simulink model "assignmen4"  (R2017a)
settings: Solver=VariableStepAuto  StartTime=0.0  StopTime=10.0  RelTol=1e-3
libraries: simulink x12, hdlsllib x12
settings Model: Creator=zhao.yi4  LastModifiedBy=yaleduffy
settings OptimizationCC: BlockReduction=off  ConditionallyExecuteInputs=off  DefaultParameterBehavior=Inlined
settings DebuggingCC: AlgebraicLoopMsg=error
settings HardwareCC: ProdBitPerPointer=32  ProdBitPerSizeT=32  ProdBitPerPtrDiffT=32  ProdLargestAtomicFloat=None  ProdIntDivRoundTo=Undefined  ProdEndianess=Unspecified  ProdWordSize=32  ProdHWDeviceType=ASIC/FPGA->ASIC/FPGA  ProdEqTarget=off

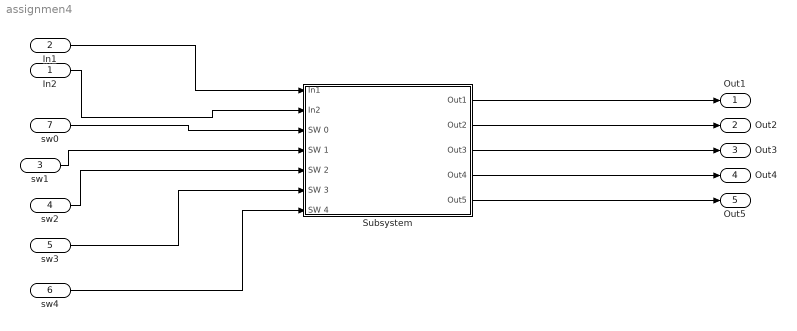
== system assignmen4 ==
  In2 : Inport  OutDataTypeStr=boolean  SampleTime=1
  In1 : Inport  Port=2  OutDataTypeStr=boolean  SampleTime=1
  sw1 : Inport  Port=3  OutDataTypeStr=boolean  SampleTime=1
  sw2 : Inport  Port=4  OutDataTypeStr=boolean  SampleTime=1
  sw3 : Inport  Port=5  OutDataTypeStr=boolean  SampleTime=1
  sw4 : Inport  Port=6  OutDataTypeStr=boolean  SampleTime=1
  sw0 : Inport  Port=7  OutDataTypeStr=boolean  SampleTime=1
  Subsystem : Subsystem
  Out1 : Outport
  Out2 : Outport  Port=2
  Out3 : Outport  Port=3
  Out4 : Outport  Port=4
  Out5 : Outport  Port=5
  wires:
  In2/1 -> Subsystem/2(In2)
  Subsystem/1(Out1) -> Out1/1
  In1/1 -> Subsystem/1(In1)
  sw2/1 -> Subsystem/5(SW 2)
  sw3/1 -> Subsystem/6(SW 3)
  sw4/1 -> Subsystem/7(SW 4)
  sw1/1 -> Subsystem/4(SW 1)
  sw0/1 -> Subsystem/3(SW 0)
  Subsystem/2(Out2) -> Out2/1
  Subsystem/3(Out3) -> Out3/1
  Subsystem/4(Out4) -> Out4/1
  Subsystem/5(Out5) -> Out5/1

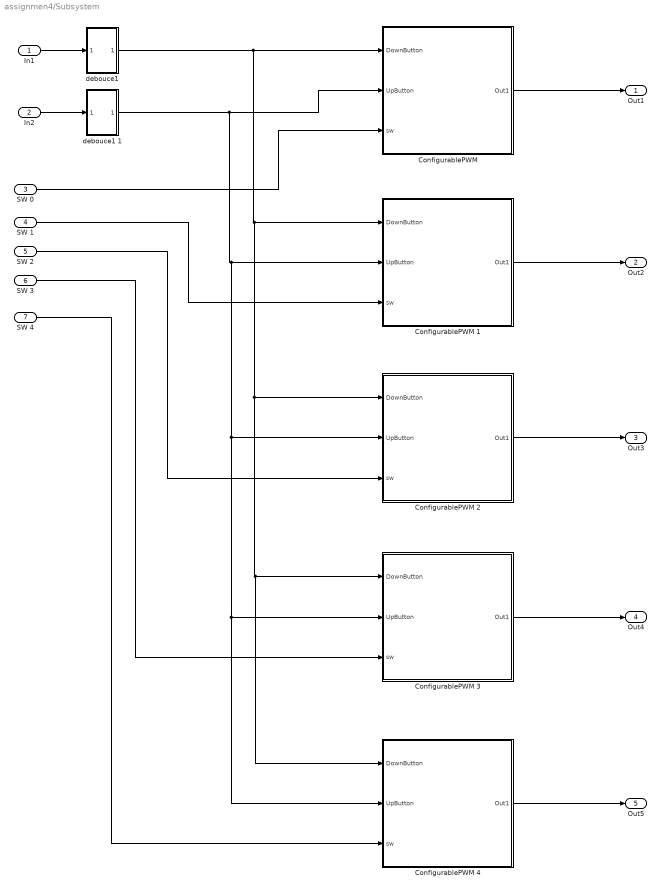
== system assignmen4/Subsystem ==
  In1 : Inport  OutDataTypeStr=boolean  SampleTime=1
  In2 : Inport  Port=2  OutDataTypeStr=boolean  SampleTime=1
  SW 0 : Inport  Port=3  OutDataTypeStr=boolean  SampleTime=1
  SW 1 : Inport  Port=4  OutDataTypeStr=boolean  SampleTime=1
  SW 2 : Inport  Port=5  OutDataTypeStr=boolean  SampleTime=1
  SW 3 : Inport  Port=6  OutDataTypeStr=boolean  SampleTime=1
  SW 4 : Inport  Port=7  OutDataTypeStr=boolean  SampleTime=1
  "ConfigurablePWM " : Subsystem
  ConfigurablePWM 1 : Subsystem
  ConfigurablePWM 2 : Subsystem
  ConfigurablePWM 3 : Subsystem
  ConfigurablePWM 4 : Subsystem
  "debouce1 " : Subsystem
  debouce1 1 : Subsystem
  Out1 : Outport
  Out2 : Outport  Port=2
  Out3 : Outport  Port=3
  Out4 : Outport  Port=4
  Out5 : Outport  Port=5
  wires:
  debouce1 1/1(Out1) -> ConfigurablePWM 4/2(UpButton), ConfigurablePWM 3/2(UpButton), ConfigurablePWM 2/2(UpButton), ConfigurablePWM 1/2(UpButton), "ConfigurablePWM "/2(UpButton)
  "debouce1 "/1(Out1) -> ConfigurablePWM 4/1(DownButton), ConfigurablePWM 3/1(DownButton), ConfigurablePWM 2/1(DownButton), ConfigurablePWM 1/1(DownButton), "ConfigurablePWM "/1(DownButton)
  "ConfigurablePWM "/1(Out1) -> Out1/1
  In1/1 -> "debouce1 "/1(In1)
  In2/1 -> debouce1 1/1(In1)
  SW 0/1 -> "ConfigurablePWM "/3(sw)
  ConfigurablePWM 1/1(Out1) -> Out2/1
  SW 1/1 -> ConfigurablePWM 1/3(sw)
  ConfigurablePWM 2/1(Out1) -> Out3/1
  ConfigurablePWM 3/1(Out1) -> Out4/1
  ConfigurablePWM 4/1(Out1) -> Out5/1
  SW 2/1 -> ConfigurablePWM 2/3(sw)
  SW 4/1 -> ConfigurablePWM 4/3(sw)
  SW 3/1 -> ConfigurablePWM 3/3(sw)

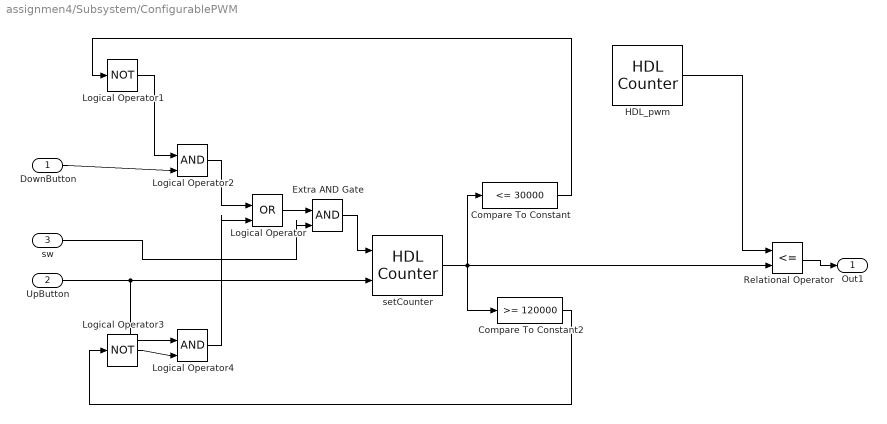
== system assignmen4/Subsystem/ConfigurablePWM  ==
  DownButton : Inport  OutDataTypeStr=boolean
  UpButton : Inport  Port=2  OutDataTypeStr=boolean
  sw : Inport  Port=3  OutDataTypeStr=boolean
  Compare To Constant : simulink/Logic and Bit Operations/Compare To Constant  relop=<=  const=30000  OutDataTypeStr=boolean
  Compare To Constant2 : simulink/Logic and Bit Operations/Compare To Constant  relop=>=  const=120000  OutDataTypeStr=boolean
  "Extra AND Gate " : Logic  IconShape=distinctive  AllPortsSameDT=off  OutDataTypeStr=boolean
  "HDL_pwm " : hdlsllib/HDL Operations/HDL Counter  CountType=Count limited  CountInit=0  CountStep=1  CountMax=1000000  CountFromType=Initial value  CountFrom=0  CountResetPort=off  CountLoadPort=off  CountEnbPort=off  CountDirPort=off  CountDataType=Unsigned  CountWordLen=32  CountFracLen=0  CountSampTime=1
      settings: SourceProductName=HDL Coder  SourceProductBaseCode=HD
  Logical Operator : Logic  Operator=OR  IconShape=distinctive  AllPortsSameDT=off  OutDataTypeStr=boolean
  Logical Operator1 : Logic  Operator=NOT  IconShape=distinctive  AllPortsSameDT=off  OutDataTypeStr=boolean
  Logical Operator2 : Logic  IconShape=distinctive  AllPortsSameDT=off  OutDataTypeStr=boolean
  Logical Operator3 : Logic  Operator=NOT  IconShape=distinctive  AllPortsSameDT=off  OutDataTypeStr=boolean
  Logical Operator4 : Logic  IconShape=distinctive  AllPortsSameDT=off  OutDataTypeStr=boolean
  Relational Operator : RelationalOperator  Operator=<=  OutDataTypeStr=boolean  RndMeth=Simplest
  setCounter : hdlsllib/HDL Operations/HDL Counter  CountType=Count limited  CountInit=75000  CountStep=6000  CountMax=120000  CountFromType=Specify  CountFrom=30000  CountResetPort=off  CountLoadPort=off  CountEnbPort=on  CountDirPort=on  CountDataType=Unsigned  CountWordLen=32  CountFracLen=0  CountSampTime=1
      settings: SourceProductName=HDL Coder  SourceProductBaseCode=HD
  Out1 : Outport  OutDataTypeStr=boolean
  wires:
  Relational Operator/1 -> Out1/1
  "HDL_pwm "/1 -> Relational Operator/1
  setCounter/1 -> Compare To Constant2/1, Relational Operator/2, Compare To Constant/1
  Compare To Constant/1 -> Logical Operator1/1
  Logical Operator2/1 -> Logical Operator/1
  Logical Operator3/1 -> Logical Operator4/2
  Logical Operator4/1 -> Logical Operator/2
  Compare To Constant2/1 -> Logical Operator3/1
  Logical Operator1/1 -> Logical Operator2/1
  DownButton/1 -> Logical Operator2/2
  UpButton/1 -> setCounter/2, Logical Operator4/1
  Logical Operator/1 -> "Extra AND Gate "/1
  sw/1 -> "Extra AND Gate "/2
  "Extra AND Gate "/1 -> setCounter/1

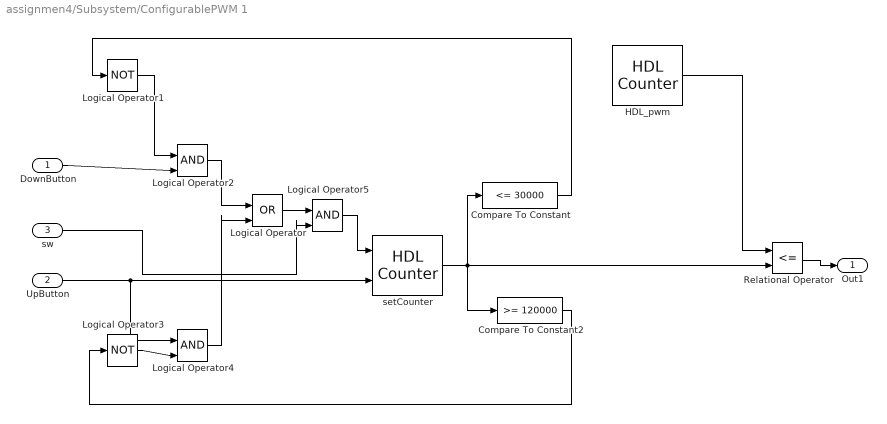
== system assignmen4/Subsystem/ConfigurablePWM 1 ==
  DownButton : Inport  OutDataTypeStr=boolean
  UpButton : Inport  Port=2  OutDataTypeStr=boolean
  sw : Inport  Port=3  OutDataTypeStr=boolean
  Compare To Constant : simulink/Logic and Bit Operations/Compare To Constant  relop=<=  const=30000  OutDataTypeStr=boolean
  Compare To Constant2 : simulink/Logic and Bit Operations/Compare To Constant  relop=>=  const=120000  OutDataTypeStr=boolean
  "HDL_pwm " : hdlsllib/HDL Operations/HDL Counter  CountType=Count limited  CountInit=0  CountStep=1  CountMax=1000000  CountFromType=Initial value  CountFrom=0  CountResetPort=off  CountLoadPort=off  CountEnbPort=off  CountDirPort=off  CountDataType=Unsigned  CountWordLen=32  CountFracLen=0  CountSampTime=1
      settings: SourceProductName=HDL Coder  SourceProductBaseCode=HD
  Logical Operator : Logic  Operator=OR  IconShape=distinctive  AllPortsSameDT=off  OutDataTypeStr=boolean
  Logical Operator1 : Logic  Operator=NOT  IconShape=distinctive  AllPortsSameDT=off  OutDataTypeStr=boolean
  Logical Operator2 : Logic  IconShape=distinctive  AllPortsSameDT=off  OutDataTypeStr=boolean
  Logical Operator3 : Logic  Operator=NOT  IconShape=distinctive  AllPortsSameDT=off  OutDataTypeStr=boolean
  Logical Operator4 : Logic  IconShape=distinctive  AllPortsSameDT=off  OutDataTypeStr=boolean
  Logical Operator5 : Logic  IconShape=distinctive  AllPortsSameDT=off  OutDataTypeStr=boolean
  Relational Operator : RelationalOperator  Operator=<=  OutDataTypeStr=boolean  RndMeth=Simplest
  setCounter : hdlsllib/HDL Operations/HDL Counter  CountType=Count limited  CountInit=75000  CountStep=6000  CountMax=120000  CountFromType=Specify  CountFrom=30000  CountResetPort=off  CountLoadPort=off  CountEnbPort=on  CountDirPort=on  CountDataType=Unsigned  CountWordLen=32  CountFracLen=0  CountSampTime=1
      settings: SourceProductName=HDL Coder  SourceProductBaseCode=HD
  Out1 : Outport  OutDataTypeStr=boolean
  wires:
  Relational Operator/1 -> Out1/1
  "HDL_pwm "/1 -> Relational Operator/1
  setCounter/1 -> Compare To Constant2/1, Relational Operator/2, Compare To Constant/1
  Compare To Constant/1 -> Logical Operator1/1
  Logical Operator2/1 -> Logical Operator/1
  Logical Operator3/1 -> Logical Operator4/2
  Logical Operator4/1 -> Logical Operator/2
  Compare To Constant2/1 -> Logical Operator3/1
  Logical Operator1/1 -> Logical Operator2/1
  DownButton/1 -> Logical Operator2/2
  UpButton/1 -> setCounter/2, Logical Operator4/1
  Logical Operator/1 -> Logical Operator5/1
  sw/1 -> Logical Operator5/2
  Logical Operator5/1 -> setCounter/1

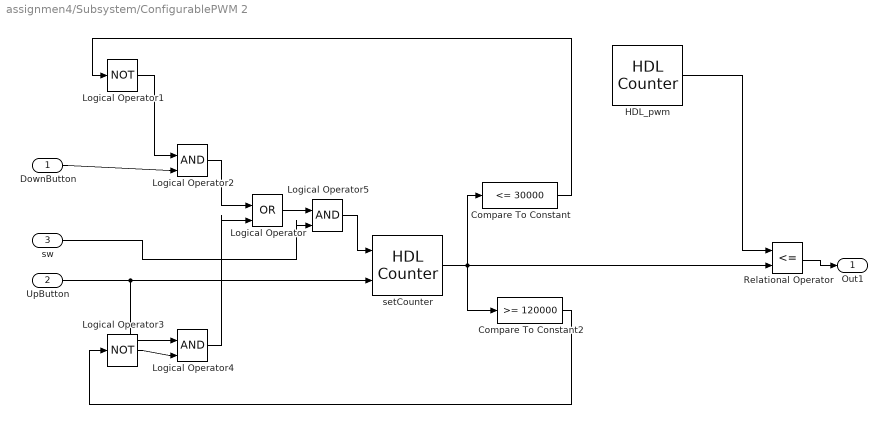
== system assignmen4/Subsystem/ConfigurablePWM 2 ==
  DownButton : Inport  OutDataTypeStr=boolean
  UpButton : Inport  Port=2  OutDataTypeStr=boolean
  sw : Inport  Port=3  OutDataTypeStr=boolean
  Compare To Constant : simulink/Logic and Bit Operations/Compare To Constant  relop=<=  const=30000  OutDataTypeStr=boolean
  Compare To Constant2 : simulink/Logic and Bit Operations/Compare To Constant  relop=>=  const=120000  OutDataTypeStr=boolean
  "HDL_pwm " : hdlsllib/HDL Operations/HDL Counter  CountType=Count limited  CountInit=0  CountStep=1  CountMax=1000000  CountFromType=Initial value  CountFrom=0  CountResetPort=off  CountLoadPort=off  CountEnbPort=off  CountDirPort=off  CountDataType=Unsigned  CountWordLen=32  CountFracLen=0  CountSampTime=1
      settings: SourceProductName=HDL Coder  SourceProductBaseCode=HD
  Logical Operator : Logic  Operator=OR  IconShape=distinctive  AllPortsSameDT=off  OutDataTypeStr=boolean
  Logical Operator1 : Logic  Operator=NOT  IconShape=distinctive  AllPortsSameDT=off  OutDataTypeStr=boolean
  Logical Operator2 : Logic  IconShape=distinctive  AllPortsSameDT=off  OutDataTypeStr=boolean
  Logical Operator3 : Logic  Operator=NOT  IconShape=distinctive  AllPortsSameDT=off  OutDataTypeStr=boolean
  Logical Operator4 : Logic  IconShape=distinctive  AllPortsSameDT=off  OutDataTypeStr=boolean
  Logical Operator5 : Logic  IconShape=distinctive  AllPortsSameDT=off  OutDataTypeStr=boolean
  Relational Operator : RelationalOperator  Operator=<=  OutDataTypeStr=boolean  RndMeth=Simplest
  setCounter : hdlsllib/HDL Operations/HDL Counter  CountType=Count limited  CountInit=75000  CountStep=6000  CountMax=120000  CountFromType=Specify  CountFrom=30000  CountResetPort=off  CountLoadPort=off  CountEnbPort=on  CountDirPort=on  CountDataType=Unsigned  CountWordLen=32  CountFracLen=0  CountSampTime=1
      settings: SourceProductName=HDL Coder  SourceProductBaseCode=HD
  Out1 : Outport  OutDataTypeStr=boolean
  wires:
  Relational Operator/1 -> Out1/1
  "HDL_pwm "/1 -> Relational Operator/1
  setCounter/1 -> Compare To Constant2/1, Relational Operator/2, Compare To Constant/1
  Compare To Constant/1 -> Logical Operator1/1
  Logical Operator2/1 -> Logical Operator/1
  Logical Operator3/1 -> Logical Operator4/2
  Logical Operator4/1 -> Logical Operator/2
  Compare To Constant2/1 -> Logical Operator3/1
  Logical Operator1/1 -> Logical Operator2/1
  DownButton/1 -> Logical Operator2/2
  UpButton/1 -> setCounter/2, Logical Operator4/1
  Logical Operator/1 -> Logical Operator5/1
  sw/1 -> Logical Operator5/2
  Logical Operator5/1 -> setCounter/1

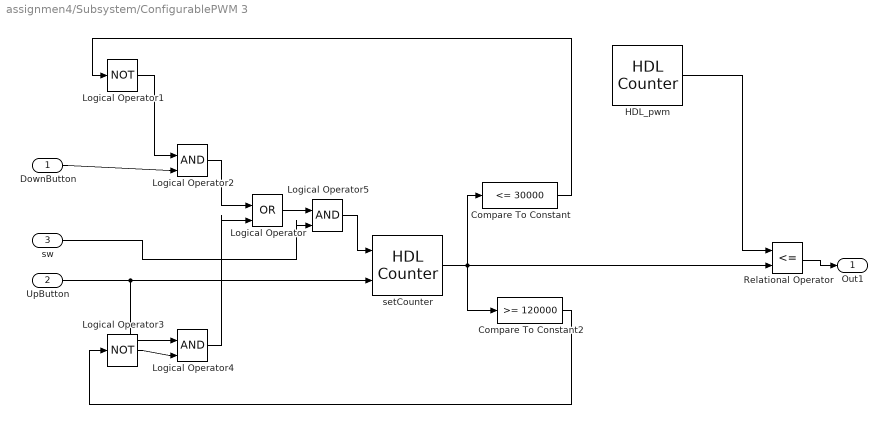
== system assignmen4/Subsystem/ConfigurablePWM 3 ==
  DownButton : Inport  OutDataTypeStr=boolean
  UpButton : Inport  Port=2  OutDataTypeStr=boolean
  sw : Inport  Port=3  OutDataTypeStr=boolean
  Compare To Constant : simulink/Logic and Bit Operations/Compare To Constant  relop=<=  const=30000  OutDataTypeStr=boolean
  Compare To Constant2 : simulink/Logic and Bit Operations/Compare To Constant  relop=>=  const=120000  OutDataTypeStr=boolean
  "HDL_pwm " : hdlsllib/HDL Operations/HDL Counter  CountType=Count limited  CountInit=0  CountStep=1  CountMax=1000000  CountFromType=Initial value  CountFrom=0  CountResetPort=off  CountLoadPort=off  CountEnbPort=off  CountDirPort=off  CountDataType=Unsigned  CountWordLen=32  CountFracLen=0  CountSampTime=1
      settings: SourceProductName=HDL Coder  SourceProductBaseCode=HD
  Logical Operator : Logic  Operator=OR  IconShape=distinctive  AllPortsSameDT=off  OutDataTypeStr=boolean
  Logical Operator1 : Logic  Operator=NOT  IconShape=distinctive  AllPortsSameDT=off  OutDataTypeStr=boolean
  Logical Operator2 : Logic  IconShape=distinctive  AllPortsSameDT=off  OutDataTypeStr=boolean
  Logical Operator3 : Logic  Operator=NOT  IconShape=distinctive  AllPortsSameDT=off  OutDataTypeStr=boolean
  Logical Operator4 : Logic  IconShape=distinctive  AllPortsSameDT=off  OutDataTypeStr=boolean
  Logical Operator5 : Logic  IconShape=distinctive  AllPortsSameDT=off  OutDataTypeStr=boolean
  Relational Operator : RelationalOperator  Operator=<=  OutDataTypeStr=boolean  RndMeth=Simplest
  setCounter : hdlsllib/HDL Operations/HDL Counter  CountType=Count limited  CountInit=75000  CountStep=6000  CountMax=120000  CountFromType=Specify  CountFrom=30000  CountResetPort=off  CountLoadPort=off  CountEnbPort=on  CountDirPort=on  CountDataType=Unsigned  CountWordLen=32  CountFracLen=0  CountSampTime=1
      settings: SourceProductName=HDL Coder  SourceProductBaseCode=HD
  Out1 : Outport  OutDataTypeStr=boolean
  wires:
  Relational Operator/1 -> Out1/1
  "HDL_pwm "/1 -> Relational Operator/1
  setCounter/1 -> Compare To Constant2/1, Relational Operator/2, Compare To Constant/1
  Compare To Constant/1 -> Logical Operator1/1
  Logical Operator2/1 -> Logical Operator/1
  Logical Operator3/1 -> Logical Operator4/2
  Logical Operator4/1 -> Logical Operator/2
  Compare To Constant2/1 -> Logical Operator3/1
  Logical Operator1/1 -> Logical Operator2/1
  DownButton/1 -> Logical Operator2/2
  UpButton/1 -> setCounter/2, Logical Operator4/1
  Logical Operator/1 -> Logical Operator5/1
  sw/1 -> Logical Operator5/2
  Logical Operator5/1 -> setCounter/1

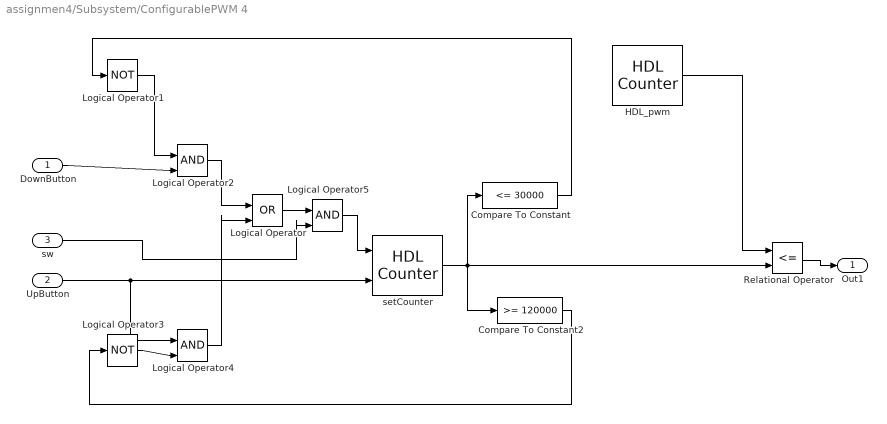
== system assignmen4/Subsystem/ConfigurablePWM 4 ==
  DownButton : Inport  OutDataTypeStr=boolean
  UpButton : Inport  Port=2  OutDataTypeStr=boolean
  sw : Inport  Port=3  OutDataTypeStr=boolean
  Compare To Constant : simulink/Logic and Bit Operations/Compare To Constant  relop=<=  const=30000  OutDataTypeStr=boolean
  Compare To Constant2 : simulink/Logic and Bit Operations/Compare To Constant  relop=>=  const=120000  OutDataTypeStr=boolean
  "HDL_pwm " : hdlsllib/HDL Operations/HDL Counter  CountType=Count limited  CountInit=0  CountStep=1  CountMax=1000000  CountFromType=Initial value  CountFrom=0  CountResetPort=off  CountLoadPort=off  CountEnbPort=off  CountDirPort=off  CountDataType=Unsigned  CountWordLen=32  CountFracLen=0  CountSampTime=1
      settings: SourceProductName=HDL Coder  SourceProductBaseCode=HD
  Logical Operator : Logic  Operator=OR  IconShape=distinctive  AllPortsSameDT=off  OutDataTypeStr=boolean
  Logical Operator1 : Logic  Operator=NOT  IconShape=distinctive  AllPortsSameDT=off  OutDataTypeStr=boolean
  Logical Operator2 : Logic  IconShape=distinctive  AllPortsSameDT=off  OutDataTypeStr=boolean
  Logical Operator3 : Logic  Operator=NOT  IconShape=distinctive  AllPortsSameDT=off  OutDataTypeStr=boolean
  Logical Operator4 : Logic  IconShape=distinctive  AllPortsSameDT=off  OutDataTypeStr=boolean
  Logical Operator5 : Logic  IconShape=distinctive  AllPortsSameDT=off  OutDataTypeStr=boolean
  Relational Operator : RelationalOperator  Operator=<=  OutDataTypeStr=boolean  RndMeth=Simplest
  setCounter : hdlsllib/HDL Operations/HDL Counter  CountType=Count limited  CountInit=75000  CountStep=6000  CountMax=120000  CountFromType=Specify  CountFrom=30000  CountResetPort=off  CountLoadPort=off  CountEnbPort=on  CountDirPort=on  CountDataType=Unsigned  CountWordLen=32  CountFracLen=0  CountSampTime=1
      settings: SourceProductName=HDL Coder  SourceProductBaseCode=HD
  Out1 : Outport  OutDataTypeStr=boolean
  wires:
  Relational Operator/1 -> Out1/1
  "HDL_pwm "/1 -> Relational Operator/1
  setCounter/1 -> Compare To Constant2/1, Relational Operator/2, Compare To Constant/1
  Compare To Constant/1 -> Logical Operator1/1
  Logical Operator2/1 -> Logical Operator/1
  Logical Operator3/1 -> Logical Operator4/2
  Logical Operator4/1 -> Logical Operator/2
  Compare To Constant2/1 -> Logical Operator3/1
  Logical Operator1/1 -> Logical Operator2/1
  DownButton/1 -> Logical Operator2/2
  UpButton/1 -> setCounter/2, Logical Operator4/1
  Logical Operator/1 -> Logical Operator5/1
  sw/1 -> Logical Operator5/2
  Logical Operator5/1 -> setCounter/1

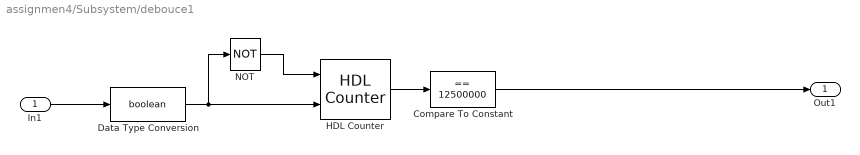
== system assignmen4/Subsystem/debouce1  ==
  In1 : Inport
  Compare To Constant : simulink/Logic and Bit Operations/Compare To Constant  relop===  const=12500000  OutDataTypeStr=boolean
  Data Type Conversion : DataTypeConversion  OutDataTypeStr=boolean
  HDL Counter : hdlsllib/HDL Operations/HDL Counter  CountType=Count limited  CountInit=0  CountStep=1  CountMax=50000000  CountFromType=Specify  CountFrom=0  CountResetPort=on  CountLoadPort=off  CountEnbPort=on  CountDirPort=off  CountDataType=Unsigned  CountWordLen=32  CountFracLen=0  CountSampTime=1
      settings: SourceProductName=HDL Coder  SourceProductBaseCode=HD
  "NOT " : Logic  Operator=NOT  IconShape=distinctive  AllPortsSameDT=off  OutDataTypeStr=boolean
  Out1 : Outport
  wires:
  Data Type Conversion/1 -> "NOT "/1, HDL Counter/2
  "NOT "/1 -> HDL Counter/1
  In1/1 -> Data Type Conversion/1
  Compare To Constant/1 -> Out1/1
  HDL Counter/1 -> Compare To Constant/1

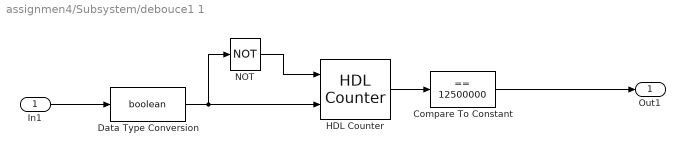
== system assignmen4/Subsystem/debouce1 1 ==
  In1 : Inport
  Compare To Constant : simulink/Logic and Bit Operations/Compare To Constant  relop===  const=12500000  OutDataTypeStr=boolean
  Data Type Conversion : DataTypeConversion  OutDataTypeStr=boolean
  HDL Counter : hdlsllib/HDL Operations/HDL Counter  CountType=Count limited  CountInit=0  CountStep=1  CountMax=50000000  CountFromType=Specify  CountFrom=0  CountResetPort=on  CountLoadPort=off  CountEnbPort=on  CountDirPort=off  CountDataType=Unsigned  CountWordLen=32  CountFracLen=0  CountSampTime=1
      settings: SourceProductName=HDL Coder  SourceProductBaseCode=HD
  "NOT " : Logic  Operator=NOT  IconShape=distinctive  AllPortsSameDT=off  OutDataTypeStr=boolean
  Out1 : Outport
  wires:
  Data Type Conversion/1 -> "NOT "/1, HDL Counter/2
  "NOT "/1 -> HDL Counter/1
  In1/1 -> Data Type Conversion/1
  Compare To Constant/1 -> Out1/1
  HDL Counter/1 -> Compare To Constant/1
